simulink model "untitled1"  (R2021a)
settings: Solver=VariableStepAuto  StartTime=0.0  StopTime=10.0  RelTol=1e-3
libraries: commdigbbndpm3 x2, commchan3 x1, commsink2 x1, commrandsrc3 x1
settings Model: Creator=soham  LastModifiedBy=soham

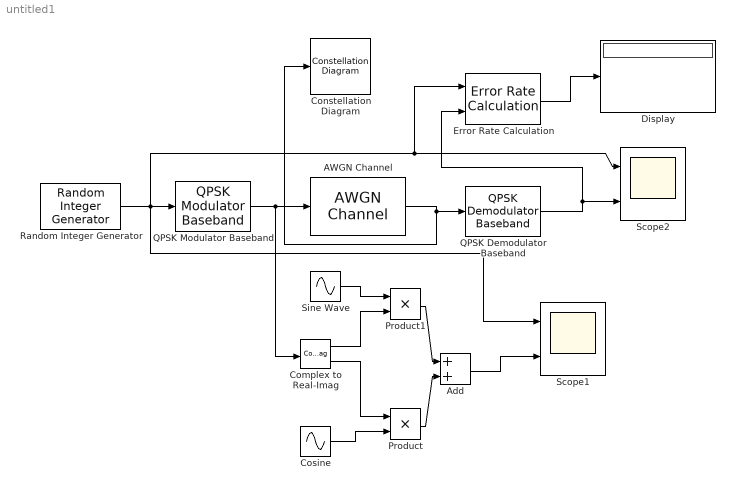
== system untitled1 ==
  AWGN Channel : commchan3/AWGN Channel  InputProcessing=Columns as channels (frame based)  seed=67  noiseMode="Signal to noise ratio  (Eb/No)"  EbNodB=10  EsNodB=10  SNRdB=10  bitsPerSym=2  Ps=1  Tsym=1  variance=1
  Add : Sum
  Complex to Real-Imag : ComplexToRealImag
  Constellation Diagram : ConstellationDiagram
  Cosine : Sin  Frequency=8*pi  Phase=pi/2  SampleTime=0.001
  Display : Display
  Error Rate Calculation : commsink2/Error Rate Calculation  N=0  st_delay=0  cp_mode=Entire frame  subframe=[]  PMode=Port  WsName=ErrorVec  RsMode2=off  stop=off  numErr=100  maxBits=1e6
  Product : Product
  Product1 : Product
  QPSK Demodulator Baseband : commdigbbndpm3/QPSK Demodulator Baseband  OutType=Integer  DecType=Hard decision  VarSource=Dialog  Variance=1  Dec=Gray  Ph=pi/4  outDtype1=Inherit via internal rule  outDtype2=Inherit via internal rule  derotateFactorWordLen=16  derotateFactorDataTypeStr=Inherit: Same word length as input  derotateFactorLastDataTypeStr=Inherit: Same word length as input
  QPSK Modulator Baseband : commdigbbndpm3/QPSK Modulator Baseband  InType=Integer  Enc=Gray  Ph=pi/4  outDtype=double  outWordLen=16  outUDDataType=sfix(16)  outFracLenMode=Best precision  outFracLen=15  outDataTypeStr=double  outLastDataTypeStr=double
  Random Integer Generator : commrandsrc3/Random Integer Generator  SetSize=8  SeedSource=Auto  Seed=0  SampleTime=1  SamplesPerFrame=1  OutputDataType=double  SimulateUsing=Interpreted execution
  Scope1 : Scope  NumInputPorts=2
  Scope2 : Scope  NumInputPorts=2
  Sine Wave : Sin  Frequency=8*pi  SampleTime=0.001
  wires:
  Add/1 -> Scope1/2
  Sine Wave/1 -> Product1/1
  Product1/1 -> Add/1
  Product/1 -> Add/2
  AWGN Channel/1 -> Constellation Diagram/1, QPSK Demodulator Baseband/1
  Cosine/1 -> Product/2
  QPSK Demodulator Baseband/1 -> Scope2/2, Error Rate Calculation/2
  Complex to Real-Imag/1 -> Product1/2
  Error Rate Calculation/1 -> Display/1
  QPSK Modulator Baseband/1 -> Complex to Real-Imag/1, AWGN Channel/1
  Complex to Real-Imag/2 -> Product/1
  Random Integer Generator/1 -> Scope1/1, Scope2/1, Error Rate Calculation/1, QPSK Modulator Baseband/1
